simulink model "UoB_Example"  (R2017a)
settings: Solver=ode3  StartTime=0.0  StopTime=90  FixedStep=0.02  RelTol=1e-3  EnableMultiTasking=on
undefined symbols (not defined in the file or in its folder): control, data
libraries: simulink x12
settings Model: SimulationMode=accelerator  Creator=Owen  LastModifiedBy=el15897
settings DataIOCC: LimitDataPoints=on  SaveFormat=Array
settings OptimizationCC: EfficientMapNaN2IntZero=off  LifeSpan=inf  AccelVerboseBuild=on
settings DebuggingCC: SolverPrmCheckMsg=warning  SFUnexpectedBacktrackingDiag=warning  SFNoUnconditionalDefaultTransitionDiag=warning  SFExecutionAtInitializationDiag=none
settings HardwareCC: ProdBitPerPointer=32  ProdBitPerSizeT=32  ProdBitPerPtrDiffT=32  ProdLargestAtomicFloat=None  ProdIntDivRoundTo=Undefined  ProdEndianess=Unspecified  ProdWordSize=32  ProdHWDeviceType=32-bit Generic  TargetBitPerPointer=64  TargetBitPerSizeT=64  TargetBitPerPtrDiffT=64  TargetLongLongMode=on  TargetIntDivRoundTo=Zero  TargetEndianess=LittleEndian  TargetWordSize=64  TargetHWDeviceType=MATLAB Host  ProdEqTarget=off
settings ModelReferenceCC: PropagateSignalLabelsOutOfModel=off
settings SFSimCC: SimCustomInitializer=initTORCSLink();  SimCustomTerminator=terminateTORCSLink();  SimUserSources=TORCSLink.c  SimBuildMode=sf_nonincremental_build  SimGenImportedTypeDefs=on
settings CodeAppCC: MaxIdLength=128
settings GRTTargetCC: TargetLangStandard=C89/C90 (ANSI)  CombineOutputUpdateFcns=off  GRTInterface=on
settings ConfigComp: CovMetricSettings=dw  CovHtmlReporting=on  CovSaveCumulativeToWorkspaceVar=on  CovSaveSingleToWorkspaceVar=on  CovExternalEMLEnable=off  CovSFcnEnable=off

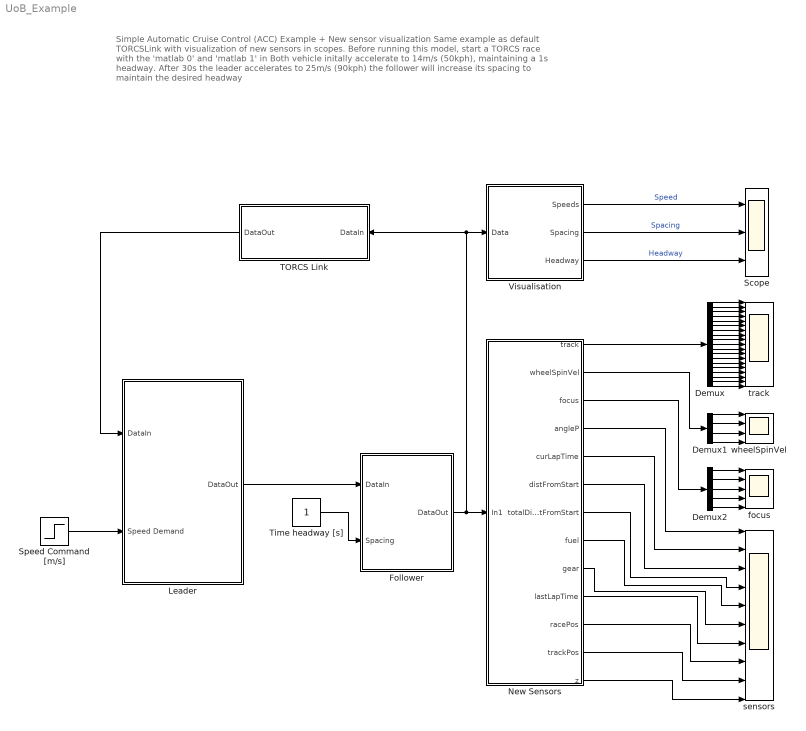
== system UoB_Example ==
  note: Simple Automatic Cruise Control (ACC) Example
      | +
      | New sensor visualization
      |
      | Same example as default TORCSLink with visualization of new sensors in scopes.
      | Before running this model, start a TORCS race with the 'matlab 0' and 'matlab 1' in
      |
      | Both vehicle initally accelerate to 14m/s (50kph), maintaining a 1s headway.
      | After 30s the leader accelerates to 25m/s (90kph)
      | the follower will increase its spacing to maintain the desired headway
  Demux : Demux  Outputs=19
  Demux1 : Demux
  Demux2 : Demux  Outputs=5
  Follower : Subsystem
      settings: CopyFcn=|
      | veh = str2num(get_param(gcb, 'vehicle'));
      | veh = veh + 1;
      | set_param(gcb,'vehicle',num2str(veh));
  Leader : Subsystem
  New Sensors : Subsystem
  Scope : Scope  NumInputPorts=3
  Speed Command [m/s] : Step  Time=30  Before=14  After=25  SampleTime=0
  TORCS Link : Subsystem  LoadFcn=|  InitFcn=|
      LoadFcn=|
      | load VehicleBusses.mat;
      | src = 'TORCSLink.c';
      | init = 'initTORCSLink();';
      | term = 'terminateTORCSLink();';
      | simSrc = get_param(gcs,'SimUserSources');
      | simInit = get_param(gcs,'SimCustomInitializer');
      | simTerm = get_param(gcs,'SimCustomTerminator');
      | 
      | if isempty(strfind(simSrc,src))
      |   fprintf('Adding %s to Custom Sources\n', src);
      |   set_param(gcs,'SimUserSources', [simSrc 10 src]);
      | end
      | 
      | if isempty(strfind(simInit,init))
      |   fprintf('Adding %s to Custom Initialisation Code\n', init);
      |   set_param(gcs,'SimCustomInitializer', [simInit 10 init]);
      | end
      | 
      | if isempty(strfind(simTerm,term))
      |   fprintf('Adding %s to Custom Termination Code\n', term);
      |   set_param(gcs,'SimCustomTerminator', [simTerm 10 term]);
      | end
      | 
      | if isunix
      |     libs = 'librt.so';
      |     simLibs = get_param(gcs,'SimUserLibraries');
      | 
      |     if isempty(strfind(simLibs,libs))
      |       fprintf('Adding %s to Custom Libraries\n', libs);
      |       set_param(gcs,'SimUserLibraries', [simLibs 10 libs]);
      |     end
      | else
      |    set_param(gcs,'SimUserLibraries', '');
      | end
      | 
      | clear src init term simSrc simInit simTerm libs simLibs;
      InitFcn=|
      | load VehicleBusses.mat;
      | src = 'TORCSLink.c';
      | init = 'initTORCSLink();';
      | term = 'terminateTORCSLink();';
      | simSrc = get_param(gcs,'SimUserSources');
      | simInit = get_param(gcs,'SimCustomInitializer');
      | simTerm = get_param(gcs,'SimCustomTerminator');
      | 
      | if isempty(strfind(simSrc,src))
      |   fprintf('Adding %s to Custom Sources\n', src);
      |   set_param(gcs,'SimUserSources', [simSrc 10 src]);
      | end
      | 
      | if isempty(strfind(simInit,init))
      |   fprintf('Adding %s to Custom Initialisation Code\n', init);
      |   set_param(gcs,'SimCustomInitializer', [simInit 10 init]);
      | end
      | 
      | if isempty(strfind(simTerm,term))
      |   fprintf('Adding %s to Custom Termination Code\n', term);
      |   set_param(gcs,'SimCustomTerminator', [simTerm 10 term]);
      | end
      | 
      | if isunix
      |     libs = 'librt.so';
      |     simLibs = get_param(gcs,'SimUserLibraries');
      | 
      |     if isempty(strfind(simLibs,libs))
      |       fprintf('Adding %s to Custom Libraries\n', libs);
      |       set_param(gcs,'SimUserLibraries', [simLibs 10 libs]);
      |     end
      | else
      |    set_param(gcs,'SimUserLibraries', '');
      | end
      | 
      | clear src init term simSrc simInit simTerm libs simLibs;
  Time headway [s] : Constant
  Visualisation : Subsystem
  focus : Scope  NumInputPorts=5
  sensors : Scope  NumInputPorts=10
  track : Scope  NumInputPorts=19
  wheelSpinVel : Scope  NumInputPorts=4
  wires:
  Leader/1(DataOut) -> Follower/1(DataIn)
  TORCS Link/1(DataOut) -> Leader/1(DataIn)
  Follower/1(DataOut) -> TORCS Link/1(DataIn), Visualisation/1(Data), New Sensors/1(In1)
  Time headway [s]/1 -> Follower/2(Spacing)
  Speed Command [m/s]/1 -> Leader/2(Speed Demand)
  Visualisation/1(Speeds) -> Scope/1  "Speed"
  Visualisation/2(Spacing) -> Scope/2  "Spacing"
  Visualisation/3(Headway) -> Scope/3  "Headway"
  New Sensors/13(z) -> sensors/10
  New Sensors/12(trackPos) -> sensors/9
  New Sensors/11(racePos) -> sensors/8
  New Sensors/10(lastLapTime) -> sensors/7
  New Sensors/9(gear) -> sensors/6
  New Sensors/8(fuel) -> sensors/5
  New Sensors/7(totalDistFromStart) -> sensors/4
  New Sensors/6(distFromStart) -> sensors/3
  New Sensors/5(curLapTime) -> sensors/2
  New Sensors/4(angleP) -> sensors/1
  New Sensors/3(focus) -> Demux2/1
  New Sensors/2(wheelSpinVel) -> Demux1/1
  New Sensors/1(track) -> Demux/1
  Demux/19 -> track/19
  Demux/18 -> track/18
  Demux/16 -> track/16
  Demux/17 -> track/17
  Demux/15 -> track/15
  Demux/13 -> track/13
  Demux/14 -> track/14
  Demux/12 -> track/12
  Demux/9 -> track/9
  Demux/10 -> track/10
  Demux/11 -> track/11
  Demux/8 -> track/8
  Demux/7 -> track/7
  Demux/6 -> track/6
  Demux/5 -> track/5
  Demux/4 -> track/4
  Demux/3 -> track/3
  Demux/2 -> track/2
  Demux/1 -> track/1
  Demux1/4 -> wheelSpinVel/4
  Demux1/3 -> wheelSpinVel/3
  Demux1/2 -> wheelSpinVel/2
  Demux1/1 -> wheelSpinVel/1
  Demux2/5 -> focus/5
  Demux2/4 -> focus/4
  Demux2/3 -> focus/3
  Demux2/2 -> focus/2
  Demux2/1 -> focus/1

== system UoB_Example/Follower ==
  note: Use a Selector block to choose which vehicle data you want,
      | then use an Assignment to overwrite that vehicles data when you're done...
  DataIn : Inport
  Spacing : Inport  Port=2
  Assignment : Assignment  DiagnosticForDimensions=Warning  IndexOptions=Index vector (dialog)  Indices=2  OutputSizes=1
  Ego : Selector  InputPortWidth=10  IndexOptions=Index vector (dialog)  Indices=2  OutputSizes=1
  Follower Vehicle Control : Subsystem
  Leader : Selector  InputPortWidth=10  IndexOptions=Index vector (dialog)  Indices=1  OutputSizes=1
  DataOut : Outport
  wires:
  Ego/1 -> Follower Vehicle Control/3(Ego)
  DataIn/1 -> Ego/1, Leader/1, Assignment/1
  Assignment/1 -> DataOut/1
  Spacing/1 -> Follower Vehicle Control/1(Headway)
  Follower Vehicle Control/1(Data Out) -> Assignment/2
  Leader/1 -> Follower Vehicle Control/2(Leader)

== system UoB_Example/Leader ==
  note: Use a Selector block to choose which vehicle data you want,
      | then use an Assignment to overwrite that vehicles data when you're done...
  DataIn : Inport
  Speed Demand : Inport  Port=2
  Assignment : Assignment  DiagnosticForDimensions=Warning  IndexOptions=Index vector (dialog)  Indices=1  OutputSizes=1
  Lead Vehicle Control : Subsystem
  Selector : Selector  InputPortWidth=10  IndexOptions=Index vector (dialog)  Indices=1  OutputSizes=1
  DataOut : Outport
  wires:
  Speed Demand/1 -> Lead Vehicle Control/2(Speed Demand)
  DataIn/1 -> Selector/1, Assignment/1
  Selector/1 -> Lead Vehicle Control/1(Data In)
  Assignment/1 -> DataOut/1
  Lead Vehicle Control/1(Data Out) -> Assignment/2

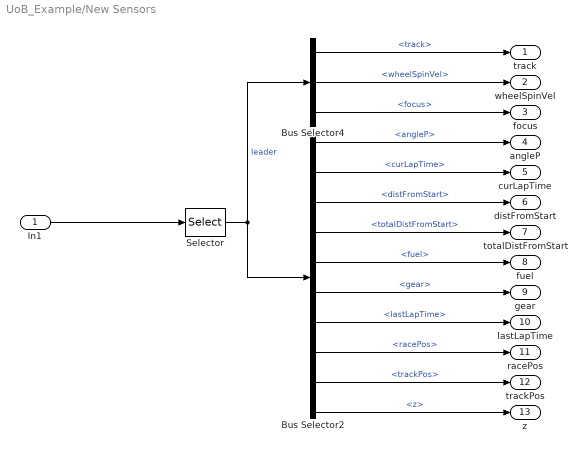
== system UoB_Example/New Sensors ==
  In1 : Inport
  Bus Selector2 : BusSelector  OutputSignals=data.angleP,data.curLapTime,data.distFromStart,data.totalDistFromStart,data.fuel,data.gear,data.lastLapTime,data.racePos,data.trackPos,data.z
  Bus Selector4 : BusSelector  OutputSignals=data.track,data.wheelSpinVel,data.focus
  Selector : Selector  InputPortWidth=10  IndexOptions=Index vector (dialog)  Indices=1  OutputSizes=1
  track : Outport
  wheelSpinVel : Outport  Port=2
  focus : Outport  Port=3
  angleP : Outport  Port=4
  curLapTime : Outport  Port=5
  distFromStart : Outport  Port=6
  totalDistFromStart : Outport  Port=7
  fuel : Outport  Port=8
  gear : Outport  Port=9
  lastLapTime : Outport  Port=10
  racePos : Outport  Port=11
  trackPos : Outport  Port=12
  z : Outport  Port=13
  wires:
  Bus Selector2/5 -> fuel/1  "<fuel>"
  Bus Selector2/10 -> z/1  "<z>"
  Bus Selector2/9 -> trackPos/1  "<trackPos>"
  Bus Selector2/8 -> racePos/1  "<racePos>"
  Bus Selector2/3 -> distFromStart/1  "<distFromStart>"
  Bus Selector4/1 -> track/1  "<track>"
  Bus Selector2/4 -> totalDistFromStart/1  "<totalDistFromStart>"
  In1/1 -> Selector/1
  Bus Selector2/6 -> gear/1  "<gear>"
  Bus Selector2/7 -> lastLapTime/1  "<lastLapTime>"
  Bus Selector2/1 -> angleP/1  "<angleP>"
  Selector/1 -> Bus Selector4/1, Bus Selector2/1  "leader"
  Bus Selector2/2 -> curLapTime/1  "<curLapTime>"
  Bus Selector4/2 -> wheelSpinVel/1  "<wheelSpinVel>"
  Bus Selector4/3 -> focus/1  "<focus>"

== system UoB_Example/TORCS Link ==
  DataIn : Inport
  FOHs : Subsystem  TreatAsAtomicUnit=on
  Memory : Memory
  Stop Simulation : Stop
  TORCSLink : MATLAB Function  TreatAsAtomicUnit=on
  DataOut : Outport
  wires:
  Memory/1 -> TORCSLink/1(vehicleDataIn)
  TORCSLink/1(vehicleDataOut) -> FOHs/1(In1)
  FOHs/1(Out1) -> DataOut/1
  DataIn/1 -> Memory/1
  TORCSLink/2(stop) -> Stop Simulation/1

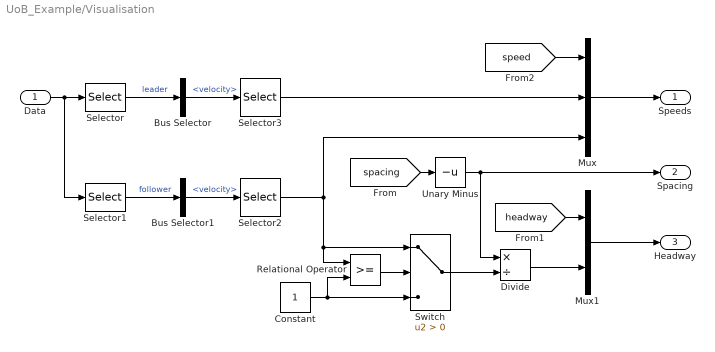
== system UoB_Example/Visualisation ==
  Data : Inport
  Bus Selector : BusSelector  OutputSignals=data.velocity
  Bus Selector1 : BusSelector  OutputSignals=data.velocity
  Constant : Constant
  Divide : Product  Inputs=*/
  Mux : Mux  Inputs=3
  Mux1 : Mux  Inputs=2
  Relational Operator : RelationalOperator  OutDataTypeStr=boolean  RndMeth=Nearest
  Selector : Selector  InputPortWidth=10  IndexOptions=Index vector (dialog)  Indices=1  OutputSizes=1
  Selector1 : Selector  InputPortWidth=10  IndexOptions=Index vector (dialog)  Indices=2  OutputSizes=1
  Selector2 : Selector  InputPortWidth=3  IndexOptions=Index vector (dialog)  Indices=1  OutputSizes=1
  Selector3 : Selector  InputPortWidth=3  IndexOptions=Index vector (dialog)  Indices=1  OutputSizes=1
  Switch : Switch  Criteria=u2 > Threshold
  Unary Minus : UnaryMinus
  Speeds : Outport
  Spacing : Outport  Port=2
  Headway : Outport  Port=3
  wires:
  Data/1 -> Selector1/1, Selector/1
  Selector/1 -> Bus Selector/1  "leader"
  Selector1/1 -> Bus Selector1/1  "follower"
  Bus Selector1/1 -> Selector2/1  "<velocity>"
  Bus Selector/1 -> Selector3/1  "<velocity>"
  Selector3/1 -> Mux/2
  Selector2/1 -> Relational Operator/1, Switch/1, Mux/3
  Mux/1 -> Speeds/1
  [spacing] -> Unary Minus/1
  Unary Minus/1 -> Divide/1, Spacing/1
  [speed] -> Mux/1
  Mux1/1 -> Headway/1
  Divide/1 -> Mux1/2
  [headway] -> Mux1/1
  Switch/1 -> Divide/2
  Relational Operator/1 -> Switch/2
  Constant/1 -> Switch/3, Relational Operator/2

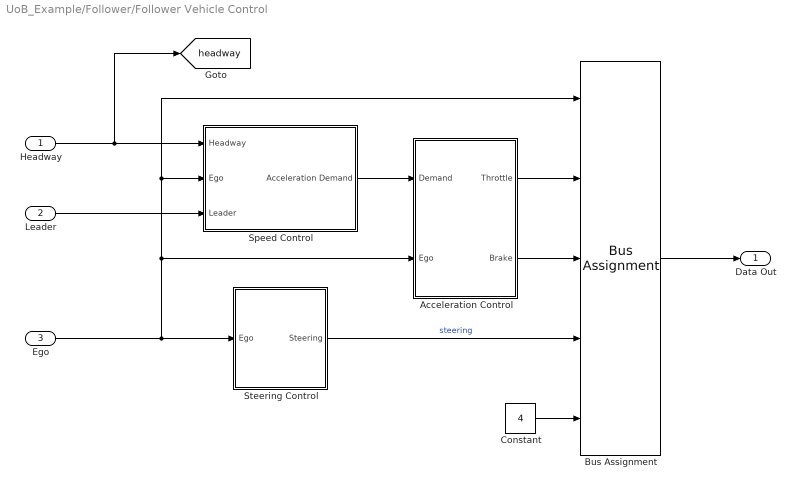
== system UoB_Example/Follower/Follower Vehicle Control ==
  Headway : Inport
  Leader : Inport  Port=2
  Ego : Inport  Port=3
  Acceleration Control : Subsystem
  Bus Assignment : BusAssignment  AssignedSignals=control.throttle,control.brake,control.steering,control.gear
  Constant : Constant  Value=4  OutDataTypeStr=int32
  Speed Control : Subsystem
  Steering Control : Subsystem
  Data Out : Outport
  tag scope: headway=global
  wires:
  Bus Assignment/1 -> Data Out/1
  Speed Control/1(Acceleration Demand) -> Acceleration Control/1(Demand)
  Headway/1 -> [headway], Speed Control/1(Headway)
  Ego/1 -> Bus Assignment/1, Speed Control/2(Ego), Acceleration Control/2(Ego), Steering Control/1(Ego)
  Leader/1 -> Speed Control/3(Leader)
  Acceleration Control/2(Brake) -> Bus Assignment/3
  Acceleration Control/1(Throttle) -> Bus Assignment/2
  Steering Control/1(Steering) -> Bus Assignment/4  "steering"
  Constant/1 -> Bus Assignment/5

== system UoB_Example/Leader/Lead Vehicle Control ==
  Data In : Inport
  Speed Demand : Inport  Port=2
  Acceleration Control : Subsystem
  Bus Assignment : BusAssignment  AssignedSignals=control.throttle,control.brake,control.steering,control.gear
  Constant : Constant  Value=4  OutDataTypeStr=int32
  Speed Control : Subsystem
  Steering Control : Subsystem
  Data Out : Outport
  tag scope: speed=global
  wires:
  Speed Demand/1 -> [speed], Speed Control/1(Demand)
  Bus Assignment/1 -> Data Out/1
  Speed Control/1(Acceleration Demand) -> Acceleration Control/1(Demand)
  Data In/1 -> Steering Control/1(Ego), Speed Control/2(Velocity), Bus Assignment/1, Acceleration Control/2(Ego)
  Acceleration Control/2(Brake) -> Bus Assignment/3
  Acceleration Control/1(Throttle) -> Bus Assignment/2
  Steering Control/1(Steering) -> Bus Assignment/4
  Constant/1 -> Bus Assignment/5

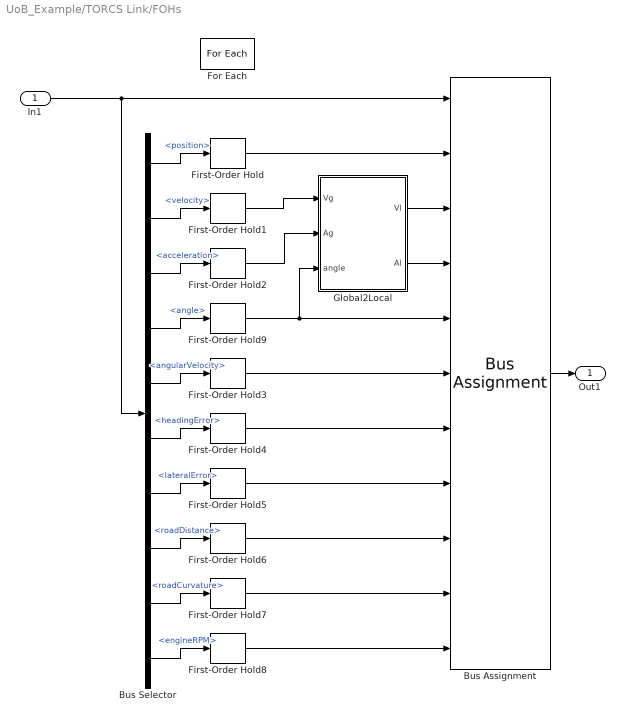
== system UoB_Example/TORCS Link/FOHs ==
  In1 : Inport  Partition=on  PartitionDimension=1  PartitionWidth=1
  Bus Assignment : BusAssignment  AssignedSignals=data.position,data.velocity,data.acceleration,data.angle,data.angularVelocity,data.headingError,data.lateralError,data.roadDistance,data.roadCurvature,data.engineRPM
  Bus Selector : BusSelector  OutputSignals=data.position,data.velocity,data.acceleration,data.angle,data.angularVelocity,data.headingError,data.lateralError,data.roadDistance,data.roadCurvature,data.engineRPM
  First-Order Hold{,1..9} (10 alike) : simulink/Discrete/First-Order Hold  DisableCoverage=on  Ts=0.02
      settings: SourceProductName=Simulink  SourceProductBaseCode=SL
  For Each : ForEach  DisableCoverage=on  IndexMode=One-based
  Global2Local : MATLAB Function  TreatAsAtomicUnit=on
  Out1 : Outport  ConcatenationDimension=1
  wires:
  Bus Assignment/1 -> Out1/1
  Bus Selector/10 -> First-Order Hold8/1  "<engineRPM>"
  Bus Selector/9 -> First-Order Hold7/1  "<roadCurvature>"
  Bus Selector/8 -> First-Order Hold6/1  "<roadDistance>"
  Bus Selector/7 -> First-Order Hold5/1  "<lateralError>"
  Bus Selector/6 -> First-Order Hold4/1  "<headingError>"
  Bus Selector/5 -> First-Order Hold3/1  "<angularVelocity>"
  Bus Selector/3 -> First-Order Hold2/1  "<acceleration>"
  Bus Selector/2 -> First-Order Hold1/1  "<velocity>"
  Bus Selector/1 -> First-Order Hold/1  "<position>"
  In1/1 -> Bus Assignment/1, Bus Selector/1
  Bus Selector/4 -> First-Order Hold9/1  "<angle>"
  First-Order Hold9/1 -> Global2Local/3(angle), Bus Assignment/5
  First-Order Hold3/1 -> Bus Assignment/6
  First-Order Hold4/1 -> Bus Assignment/7
  First-Order Hold5/1 -> Bus Assignment/8
  First-Order Hold6/1 -> Bus Assignment/9
  First-Order Hold7/1 -> Bus Assignment/10
  First-Order Hold8/1 -> Bus Assignment/11
  First-Order Hold1/1 -> Global2Local/1(Vg)
  First-Order Hold2/1 -> Global2Local/2(Ag)
  First-Order Hold/1 -> Bus Assignment/2
  Global2Local/2(Al) -> Bus Assignment/4
  Global2Local/1(Vl) -> Bus Assignment/3

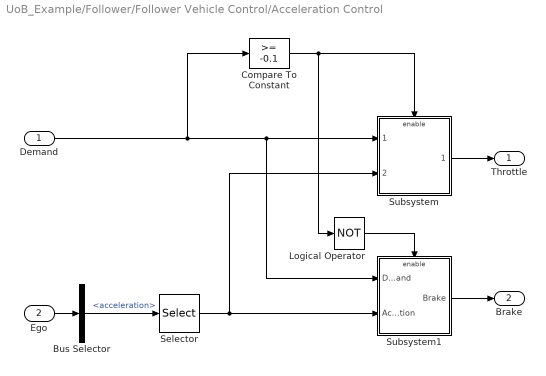
== system UoB_Example/Follower/Follower Vehicle Control/Acceleration Control ==
  Demand : Inport
  Ego : Inport  Port=2
  Bus Selector : BusSelector  OutputSignals=data.acceleration
  Compare To Constant : simulink/Logic and Bit Operations/Compare To Constant  relop=>=  const=-0.1  OutDataTypeStr=boolean
  Logical Operator : Logic  Operator=NOT  AllPortsSameDT=off  OutDataTypeStr=boolean
  Selector : Selector  InputPortWidth=3  IndexOptions=Index vector (dialog)  Indices=1  OutputSizes=1
  Subsystem : Subsystem
  Subsystem1 : Subsystem
  Throttle : Outport
  Brake : Outport  Port=2
  wires:
  Selector/1 -> Subsystem/2(Acceleration), Subsystem1/2(Acceleration)
  Demand/1 -> Compare To Constant/1, Subsystem1/1(Demand), Subsystem/1(Demand)
  Subsystem1/1(Brake) -> Brake/1
  Subsystem/1(Throttle) -> Throttle/1
  Compare To Constant/1 -> Subsystem/Enable, Logical Operator/1
  Logical Operator/1 -> Subsystem1/Enable
  Ego/1 -> Bus Selector/1
  Bus Selector/1 -> Selector/1  "<acceleration>"

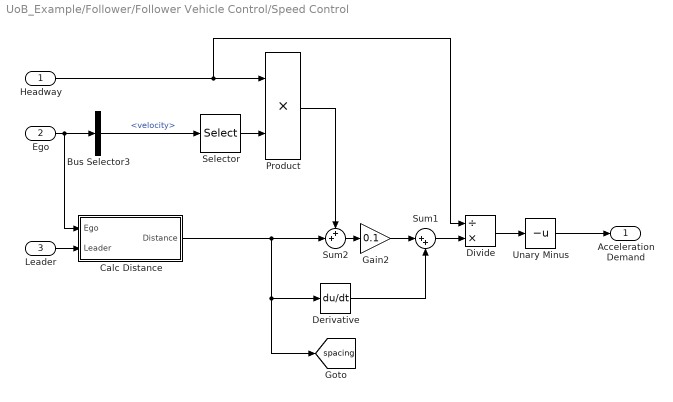
== system UoB_Example/Follower/Follower Vehicle Control/Speed Control ==
  Headway : Inport
  Ego : Inport  Port=2
  Leader : Inport  Port=3
  Bus Selector3 : BusSelector  OutputSignals=data.velocity
  Calc Distance : Subsystem
  Derivative : Derivative
  Divide : Product  Inputs=/*
  Gain2 : Gain  Gain=0.1
  Product : Product
  Selector : Selector  InputPortWidth=3  IndexOptions=Index vector (dialog)  Indices=1  OutputSizes=1
  Sum1 : Sum  Inputs=|++
  Sum2 : Sum  Inputs=++|
  Unary Minus : UnaryMinus
  Acceleration Demand : Outport
  tag scope: spacing=global
  wires:
  Ego/1 -> Calc Distance/1(Ego), Bus Selector3/1
  Leader/1 -> Calc Distance/2(Leader)
  Bus Selector3/1 -> Selector/1  "<velocity>"
  Headway/1 -> Divide/1, Product/1
  Selector/1 -> Product/2
  Calc Distance/1(Distance) -> Derivative/1, [spacing], Sum2/2
  Product/1 -> Sum2/1
  Sum2/1 -> Gain2/1
  Gain2/1 -> Sum1/1
  Derivative/1 -> Sum1/2
  Sum1/1 -> Divide/2
  Divide/1 -> Unary Minus/1
  Unary Minus/1 -> Acceleration Demand/1

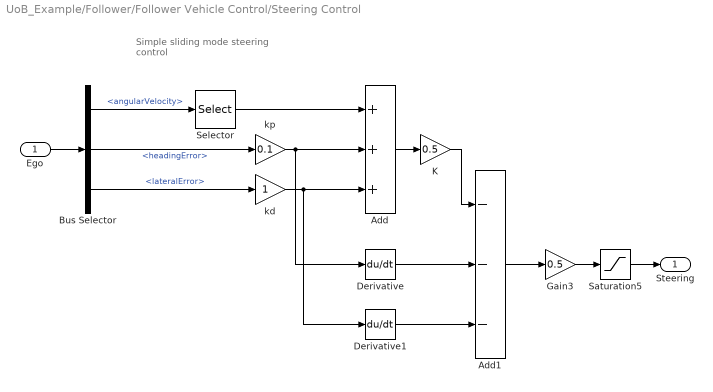
== system UoB_Example/Follower/Follower Vehicle Control/Steering Control ==
  note: Simple sliding mode steering control
  Ego : Inport
  Add : Sum  Inputs=+++
  Add1 : Sum  Inputs=---
  Bus Selector : BusSelector  OutputSignals=data.angularVelocity,data.headingError,data.lateralError
  Derivative : Derivative
  Derivative1 : Derivative
  Gain3 : Gain  Gain=0.5
  K : Gain  Gain=0.5
  Saturation5 : Saturate
  Selector : Selector  InputPortWidth=3  IndexOptions=Index vector (dialog)  Indices=3  OutputSizes=1
  kd : Gain
  kp : Gain  Gain=0.1
  Steering : Outport
  wires:
  Ego/1 -> Bus Selector/1
  Add1/1 -> Gain3/1
  K/1 -> Add1/1
  Derivative1/1 -> Add1/3
  Derivative/1 -> Add1/2
  Add/1 -> K/1
  kp/1 -> Derivative/1, Add/2
  kd/1 -> Derivative1/1, Add/3
  Bus Selector/3 -> kd/1  "<lateralError>"
  Bus Selector/2 -> kp/1  "<headingError>"
  Gain3/1 -> Saturation5/1
  Saturation5/1 -> Steering/1
  Selector/1 -> Add/1
  Bus Selector/1 -> Selector/1  "<angularVelocity>"

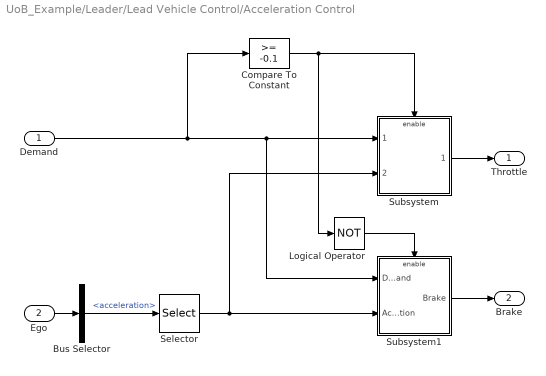
== system UoB_Example/Leader/Lead Vehicle Control/Acceleration Control ==
  Demand : Inport
  Ego : Inport  Port=2
  Bus Selector : BusSelector  OutputSignals=data.acceleration
  Compare To Constant : simulink/Logic and Bit Operations/Compare To Constant  relop=>=  const=-0.1  OutDataTypeStr=boolean
  Logical Operator : Logic  Operator=NOT  AllPortsSameDT=off  OutDataTypeStr=boolean
  Selector : Selector  InputPortWidth=3  IndexOptions=Index vector (dialog)  Indices=1  OutputSizes=1
  Subsystem : Subsystem
  Subsystem1 : Subsystem
  Throttle : Outport
  Brake : Outport  Port=2
  wires:
  Selector/1 -> Subsystem/2(Acceleration), Subsystem1/2(Acceleration)
  Demand/1 -> Compare To Constant/1, Subsystem1/1(Demand), Subsystem/1(Demand)
  Subsystem1/1(Brake) -> Brake/1
  Subsystem/1(Throttle) -> Throttle/1
  Compare To Constant/1 -> Subsystem/Enable, Logical Operator/1
  Logical Operator/1 -> Subsystem1/Enable
  Ego/1 -> Bus Selector/1
  Bus Selector/1 -> Selector/1  "<acceleration>"

== system UoB_Example/Leader/Lead Vehicle Control/Speed Control ==
  Demand : Inport
  Velocity : Inport  Port=2
  Bus Selector : BusSelector  OutputSignals=data.velocity
  Gain : Gain  Gain=0.5
  Rate Limiter : RateLimiter  RisingSlewLimit=inf  FallingSlewLimit=-inf  SampleTimeMode=inherited
  Saturation : Saturate  UpperLimit=2  LowerLimit=-4
  Selector : Selector  InputPortWidth=3  IndexOptions=Index vector (dialog)  Indices=1  OutputSizes=1
  Sum : Sum  Inputs=|+-
  Acceleration Demand : Outport
  wires:
  Gain/1 -> Saturation/1
  Sum/1 -> Gain/1
  Demand/1 -> Sum/1
  Saturation/1 -> Rate Limiter/1
  Selector/1 -> Sum/2
  Rate Limiter/1 -> Acceleration Demand/1
  Velocity/1 -> Bus Selector/1
  Bus Selector/1 -> Selector/1  "<velocity>"

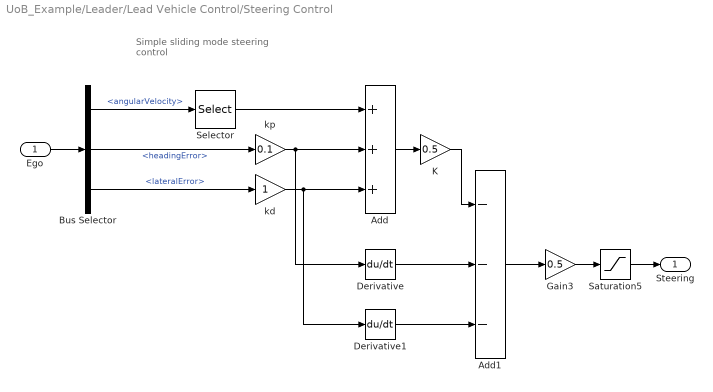
== system UoB_Example/Leader/Lead Vehicle Control/Steering Control ==
  note: Simple sliding mode steering control
  Ego : Inport
  Add : Sum  Inputs=+++
  Add1 : Sum  Inputs=---
  Bus Selector : BusSelector  OutputSignals=data.angularVelocity,data.headingError,data.lateralError
  Derivative : Derivative
  Derivative1 : Derivative
  Gain3 : Gain  Gain=0.5
  K : Gain  Gain=0.5
  Saturation5 : Saturate
  Selector : Selector  InputPortWidth=3  IndexOptions=Index vector (dialog)  Indices=3  OutputSizes=1
  kd : Gain
  kp : Gain  Gain=0.1
  Steering : Outport
  wires:
  Ego/1 -> Bus Selector/1
  Add1/1 -> Gain3/1
  K/1 -> Add1/1
  Derivative1/1 -> Add1/3
  Derivative/1 -> Add1/2
  Add/1 -> K/1
  kp/1 -> Derivative/1, Add/2
  kd/1 -> Derivative1/1, Add/3
  Bus Selector/3 -> kd/1  "<lateralError>"
  Bus Selector/2 -> kp/1  "<headingError>"
  Gain3/1 -> Saturation5/1
  Saturation5/1 -> Steering/1
  Selector/1 -> Add/1
  Bus Selector/1 -> Selector/1  "<angularVelocity>"

== system UoB_Example/Follower/Follower Vehicle Control/Acceleration Control/Subsystem ==
  Demand : Inport
  Acceleration : Inport  Port=2
  Enable : EnablePort  StatesWhenEnabling=reset
  Gain : Gain  Gain=1.5
  Gain1 : Gain  Gain=10
  Integrator Limited : Integrator  LimitOutput=on  UpperSaturationLimit=1  LowerSaturationLimit=-1
  Sum : Sum  Inputs=++|
  Sum1 : Sum  Inputs=+-|
  Throttle : Outport  OutputWhenDisabled=reset  InitialOutput=0
  wires:
  Gain/1 -> Sum/1
  Integrator Limited/1 -> Sum/2
  Gain1/1 -> Integrator Limited/1
  Sum/1 -> Throttle/1
  Demand/1 -> Sum1/1, Gain/1
  Acceleration/1 -> Sum1/2
  Sum1/1 -> Gain1/1

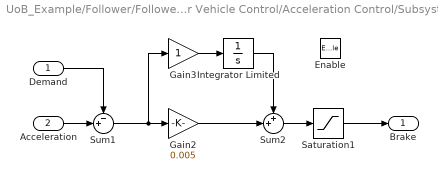
== system UoB_Example/Follower/Follower Vehicle Control/Acceleration Control/Subsystem1 ==
  Demand : Inport
  Acceleration : Inport  Port=2
  Enable : EnablePort  StatesWhenEnabling=reset
  Gain2 : Gain  Gain=0.005
  Gain3 : Gain
  Integrator Limited : Integrator  LimitOutput=on  UpperSaturationLimit=1  LowerSaturationLimit=-1
  Saturation1 : Saturate  UpperLimit=1  LowerLimit=0
  Sum1 : Sum  Inputs=-+|
  Sum2 : Sum  Inputs=++|
  Brake : Outport  OutputWhenDisabled=reset  InitialOutput=0
  wires:
  Saturation1/1 -> Brake/1
  Sum2/1 -> Saturation1/1
  Gain2/1 -> Sum2/2
  Integrator Limited/1 -> Sum2/1
  Gain3/1 -> Integrator Limited/1
  Sum1/1 -> Gain2/1, Gain3/1
  Demand/1 -> Sum1/1
  Acceleration/1 -> Sum1/2

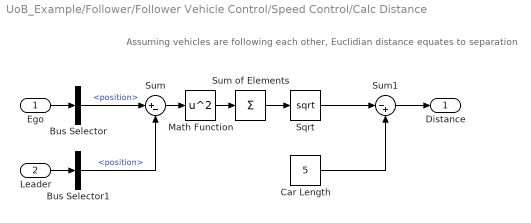
== system UoB_Example/Follower/Follower Vehicle Control/Speed Control/Calc Distance ==
  note: Assuming vehicles are following each other, Euclidian distance equates to separation
  Ego : Inport
  Leader : Inport  Port=2
  Bus Selector : BusSelector  OutputSignals=data.position
  Bus Selector1 : BusSelector  OutputSignals=data.position
  Car Length : Constant  Value=5
  Math Function : Math  Operator=square  SaturateOnIntegerOverflow=on
  Sqrt : Sqrt  SaturateOnIntegerOverflow=on
  Sum : Sum  Inputs=|+-
  Sum of Elements : Sum  Inputs=+
  Sum1 : Sum  Inputs=|-+
  Distance : Outport
  wires:
  Ego/1 -> Bus Selector/1
  Leader/1 -> Bus Selector1/1
  Bus Selector/1 -> Sum/1  "<position>"
  Bus Selector1/1 -> Sum/2  "<position>"
  Sum/1 -> Math Function/1
  Math Function/1 -> Sum of Elements/1
  Sum of Elements/1 -> Sqrt/1
  Sum1/1 -> Distance/1
  Sqrt/1 -> Sum1/1
  Car Length/1 -> Sum1/2

== system UoB_Example/Leader/Lead Vehicle Control/Acceleration Control/Subsystem ==
  Demand : Inport
  Acceleration : Inport  Port=2
  Enable : EnablePort  StatesWhenEnabling=reset
  Gain : Gain  Gain=1.5
  Gain1 : Gain  Gain=10
  Integrator Limited : Integrator  LimitOutput=on  UpperSaturationLimit=1  LowerSaturationLimit=-1
  Sum : Sum  Inputs=++|
  Sum1 : Sum  Inputs=+-|
  Throttle : Outport  OutputWhenDisabled=reset  InitialOutput=0
  wires:
  Gain/1 -> Sum/1
  Integrator Limited/1 -> Sum/2
  Gain1/1 -> Integrator Limited/1
  Sum/1 -> Throttle/1
  Demand/1 -> Sum1/1, Gain/1
  Acceleration/1 -> Sum1/2
  Sum1/1 -> Gain1/1

== system UoB_Example/Leader/Lead Vehicle Control/Acceleration Control/Subsystem1 ==
  Demand : Inport
  Acceleration : Inport  Port=2
  Enable : EnablePort  StatesWhenEnabling=reset
  Gain2 : Gain  Gain=0.005
  Gain3 : Gain
  Integrator Limited : Integrator  LimitOutput=on  UpperSaturationLimit=1  LowerSaturationLimit=-1
  Saturation1 : Saturate  UpperLimit=1  LowerLimit=0
  Sum1 : Sum  Inputs=-+|
  Sum2 : Sum  Inputs=++|
  Brake : Outport  OutputWhenDisabled=reset  InitialOutput=0
  wires:
  Saturation1/1 -> Brake/1
  Sum2/1 -> Saturation1/1
  Gain2/1 -> Sum2/2
  Integrator Limited/1 -> Sum2/1
  Gain3/1 -> Integrator Limited/1
  Sum1/1 -> Gain2/1, Gain3/1
  Demand/1 -> Sum1/1
  Acceleration/1 -> Sum1/2

== matlab function UoB_Example/TORCS Link/TORCSLink ==
  data: vehicleDataIn input Bus: VehicleBus size=10; vehicleDataOut output Bus: VehicleBus size=10; stop output
function [vehicleDataOut, stop] = TORCSLink(vehicleDataIn)
%#codegen
stop = 0;
flag = int32(0);

% Simulink doesn't like passing the array of structures to C function (no
% idea why?!), so we have to seperate out the three stages

% Update vehicle control values in TORCS
for i=1:10
    flag = coder.ceval('setVehicleControl', int32(i-1), vehicleDataIn(i).control);
    if (flag < 0)
        fprintf('No connection to TORCS!\n');
        stop = 1;
    end
end

% Tell TORCS it can update (this function hangs until new data is
% available)
flag = coder.ceval('updateTORCS');
if (flag < 0)
    fprintf('No data from TORCS! (%d) \n', flag);
    stop = 1;
end

% Read in new data from TORCS
for i=1:10
    % Can't pass this directly to coder.ref
    data = vehicleDataIn(i).data;
    flag = coder.ceval('getVehicleData', int32(i-1), coder.ref(data));
    vehicleDataIn(i).data = data;
    if (flag < 0)
        fprintf('No connection to TORCS!\n');
        stop = 1;
    end
end

vehicleDataOut = vehicleDataIn;

== matlab function UoB_Example/TORCS Link/FOHs/Global2Local ==
  data: Vg input; Ag input; angle input; Vl output; Al output
function [Vl,Al] = fcn(Vg,Ag,angle)
%#codegen

phi=angle(3);
R = [cos(phi) sin(phi) 0; -sin(phi) cos(phi) 0; 0 0 1];

Vl = R*Vg;
Al = R*Ag;
